simulink subsystem "battery_module"  (R2021a)
settings: Solver=VariableStepAuto  StartTime=0.0  StopTime=10.0  RelTol=1e-3
undefined symbols (not defined in the file): InitialAmbientTemperature
libraries: fl_lib x4, nesl_utility x3
settings Model: Creator=Carlo Edoardo  LastModifiedBy=Carlo Edoardo

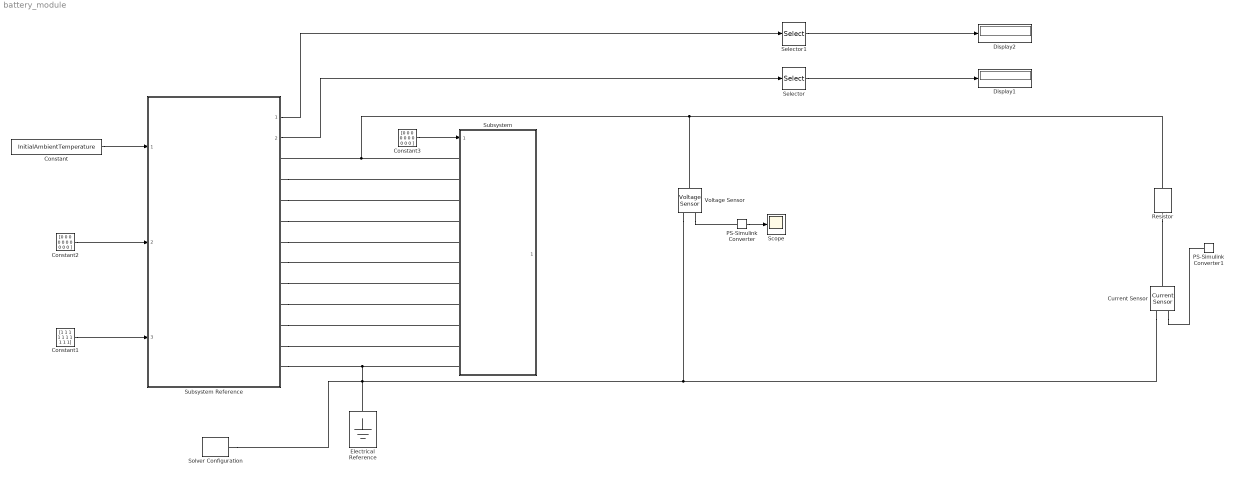
== system battery_module ==
  Constant : Constant  Value=InitialAmbientTemperature
  Constant1 : Constant  Value=[1 1 1 1 1 1 1 1 1 1]
  Constant2 : Constant  Value=[0 0 0 0 0 0 0 0 0 0 ]
  Constant3 : Constant  Value=[0 0 0 0 0 0 0 0 0 0 ]
  Current Sensor : fl_lib/Electrical/Electrical Sensors/Current Sensor
  Display1 : Display
  Display2 : Display
  Electrical Reference : fl_lib/Electrical/Electrical Elements/Electrical Reference
  PS-Simulink Converter : nesl_utility/PS-Simulink Converter  PhysicalDomain=network_engine_domain  SubClassName=ps_output  LeftPortType=input  RightPortType=output  PseudoPeriodic=off  Frequencies=[]  Unit=inherit  AffineConversion=off
      settings: SourceProductBaseCode=PW,SS
  PS-Simulink Converter1 : nesl_utility/PS-Simulink Converter  PhysicalDomain=network_engine_domain  SubClassName=ps_output  LeftPortType=input  RightPortType=output  PseudoPeriodic=off  Frequencies=[]  Unit=inherit  AffineConversion=off
      settings: SourceProductBaseCode=PW,SS
  Resistor : fl_lib/Electrical/Electrical Elements/Resistor  R=0.1 Ohm  i_specify=off  i_priority=None  i=0 A  i_nominal_specify=off  i_nominal_unit=A  i_nominal_value=1  v_specify=off  v_priority=None  v=0 V  v_nominal_specify=off  v_nominal_unit=V  v_nominal_value=1
  Scope : Scope
  Selector : Selector  InputPortWidth=10  IndexOptions=Index vector (dialog)  Indices=1  OutputSizes=1
  Selector1 : Selector  InputPortWidth=10  IndexOptions=Index vector (dialog)  Indices=1  OutputSizes=1
  Solver Configuration : nesl_utility/Solver Configuration  PhysicalDomain=network_engine_domain  SubClassName=solver  LeftPortType=input  RightPortType=generic  Tones=[]  Harmonics=[]  SimulateNoise=off  Profile=off  UseLocalSampling=off  EnableSwitchedLinearOptims=on  FrequencyDomain=off  UseCCode=off  RelTol=0.001  AbsTol=1e-06  MinStep=1e-09  ToWorkspace=off  RevertToSquareIcSolve=off  NumHomotopyIterations=100  PhasorMode=off  PhasorModeNumHarmonics=1  DoDC=off  ResidualTolerance=1e-09  UseLocalSolver=on  LocalSolverChoice=NE_BACKWARD_EULER_ADVANCER  LocalSolverSampleTime=0.001  DoFixedCost=on  MaxNonlinIter=3  MaxModeIter=2  ComputeImpulses=off  ImpulseIterations=2  LinearAlgebra=auto  EquationFormulation=NE_TIME_EF  DelaysMemoryBudget=1024  AutomaticFiltering=on  FilteringTimeConstant=0.001  PartitionStorageMethod=AS_NEEDED  PartitionMemoryBudget=1024  PartitionMethod=ROBUST
      settings: SourceProductBaseCode=PW,SS
  Subsystem : Subsystem  ReferencedSubsystem=BMS_slave
  Subsystem Reference : Subsystem  ReferencedSubsystem=battery_segment
  Voltage Sensor : fl_lib/Electrical/Electrical Sensors/Voltage Sensor
  wires:
  Constant/1 -> Subsystem Reference/1
  Subsystem Reference/2 -> Selector/1
  Selector/1 -> Display1/1
  Selector1/1 -> Display2/1
  Subsystem Reference/1 -> Selector1/1
  Constant1/1 -> Subsystem Reference/3
  Constant2/1 -> Subsystem Reference/2
  PS-Simulink Converter/1 -> Scope/1
  Constant3/1 -> Subsystem/1
  connections:
  Voltage Sensor/RConn2 -- Current Sensor/RConn2 -- Solver Configuration/RConn1 -- Electrical Reference/LConn1 -- Subsystem/LConn11 -- Subsystem Reference/RConn11
  Resistor/LConn1 -- Voltage Sensor/LConn1 -- Subsystem Reference/RConn1 -- Subsystem/LConn1
  Subsystem Reference/RConn2 -- Subsystem/LConn2
  Subsystem Reference/RConn3 -- Subsystem/LConn3
  Subsystem Reference/RConn4 -- Subsystem/LConn4
  Subsystem Reference/RConn5 -- Subsystem/LConn5
  Subsystem Reference/RConn6 -- Subsystem/LConn6
  Subsystem Reference/RConn7 -- Subsystem/LConn7
  Subsystem Reference/RConn8 -- Subsystem/LConn8
  Subsystem Reference/RConn9 -- Subsystem/LConn9
  Subsystem Reference/RConn10 -- Subsystem/LConn10
  Voltage Sensor/RConn1 -- PS-Simulink Converter/LConn1
  Resistor/RConn1 -- Current Sensor/LConn1
  Current Sensor/RConn1 -- PS-Simulink Converter1/LConn1
